simulink model "ACC_simu"  (R2023a)
settings: Solver=VariableStepAuto  StartTime=0.0  StopTime=400  RelTol=1e-3
values from neighbouring files (symbols this model uses):
  amax_ego = 1.47    [ACC_code.m]
  amin_ego = -5    [ACC_code.m]
  b = 50    [ACC_code.m]
  Brake_Pedal_Sensor = 0    [ACC_code.m]
  D_default = 10    [ACC_code.m]
  Fault_signal = 0    [ACC_code.m]
  Gas_Pedal_Sensor = 0    [ACC_code.m]
  m = 1000    [ACC_code.m]
  Time_Gap = 3    [ACC_code.m]
  Ts = 0.01    [ACC_code.m]
  v0_ego = 80    [ACC_code.m]
  v0_lead = 90    [ACC_code.m]
  x0_ego = 30    [ACC_code.m]
  x0_lead = 50    [ACC_code.m]
undefined symbols (not defined in the file or in its folder): h, km, s
libraries: aerolibconvert2 x6, simulink x2
settings Model: Creator=Leo  LastModifiedBy=Usuario
settings OptimizationCC: BlockReduction=off  DefaultParameterBehavior=Inlined  BufferReuse=off

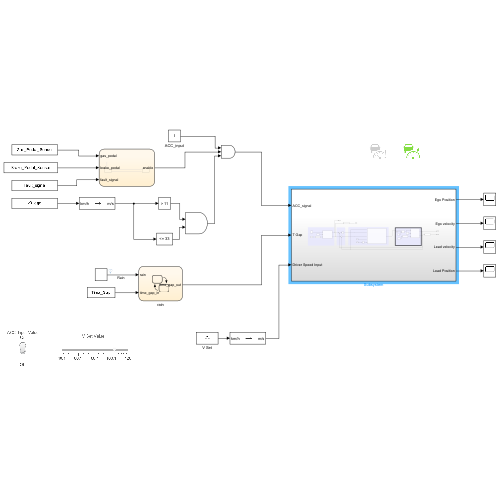
[thumbnail: Simulink's stored preview of the top-level diagram]
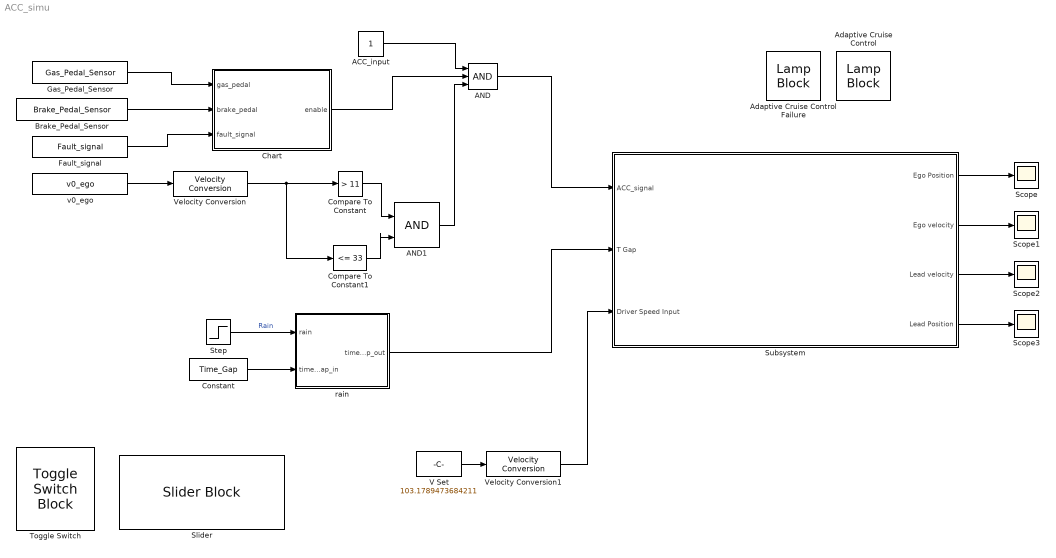
== system ACC_simu ==
  ACC_input : Constant
  AND : Logic  Inputs=3  IconShape=distinctive  AllPortsSameDT=off  OutDataTypeStr=boolean
  AND1 : Logic  IconShape=distinctive  AllPortsSameDT=off  OutDataTypeStr=boolean
  Adaptive Cruise Control : LampBlock  LabelPosition=Hide  Icon=AdaptiveCruiseControl
  Adaptive Cruise Control Failure : LampBlock  LabelPosition=Hide  Icon=AdaptiveCruiseControlFailure
  Brake_Pedal_Sensor : Constant  Value=Brake_Pedal_Sensor  SampleTime=Ts
  Chart : Stateflow chart  TreatAsAtomicUnit=on
  Compare To Constant : simulink/Logic and Bit Operations/Compare To Constant  relop=>  const=11  OutDataTypeStr=boolean
  Compare To Constant1 : simulink/Logic and Bit Operations/Compare To Constant  relop=<=  const=33  OutDataTypeStr=boolean
  Constant : Constant  Value=Time_Gap  SampleTime=Ts
  Fault_signal : Constant  Value=Fault_signal  SampleTime=Ts
  Gas_Pedal_Sensor : Constant  Value=Gas_Pedal_Sensor  SampleTime=Ts
  Scope{,1..3} (4 alike) : Scope
  Slider : SliderBlock  ScaleMin=40.1  ScaleMax=120
  Step : Step  Time=500
  Subsystem : Subsystem
  Toggle Switch : ToggleSwitchBlock
      settings: Values={{'Off', 'On'}, [0 1]}
  V Set : Constant  Value=103.1789473684211
  Velocity Conversion : aerolibconvert2/Velocity Conversion  IU=km/h  OU=m/s
  Velocity Conversion1 : aerolibconvert2/Velocity Conversion  IU=km/h  OU=m/s
  rain : Stateflow chart  TreatAsAtomicUnit=on
  v0_ego : Constant  Value=v0_ego  SampleTime=Ts
  wires:
  ACC_input/1 -> AND/1
  rain/1(time_gap_out) -> Subsystem/2(T Gap)
  Step/1 -> rain/1(rain)  "Rain"
  v0_ego/1 -> Velocity Conversion/1
  Compare To Constant/1 -> AND1/1
  Compare To Constant1/1 -> AND1/2
  AND1/1 -> AND/3
  AND/1 -> Subsystem/1(ACC_signal)
  Constant/1 -> rain/2(time_gap_in)
  Gas_Pedal_Sensor/1 -> Chart/1(gas_pedal)
  Brake_Pedal_Sensor/1 -> Chart/2(brake_pedal)
  Fault_signal/1 -> Chart/3(fault_signal)
  Chart/1(enable) -> AND/2
  Velocity Conversion/1 -> Compare To Constant1/1, Compare To Constant/1
  V Set/1 -> Velocity Conversion1/1
  Velocity Conversion1/1 -> Subsystem/3(Driver Speed Input)
  Subsystem/2(Ego velocity) -> Scope1/1
  Subsystem/1(Ego Position) -> Scope/1
  Subsystem/3(Lead velocity) -> Scope2/1
  Subsystem/4(Lead Position) -> Scope3/1

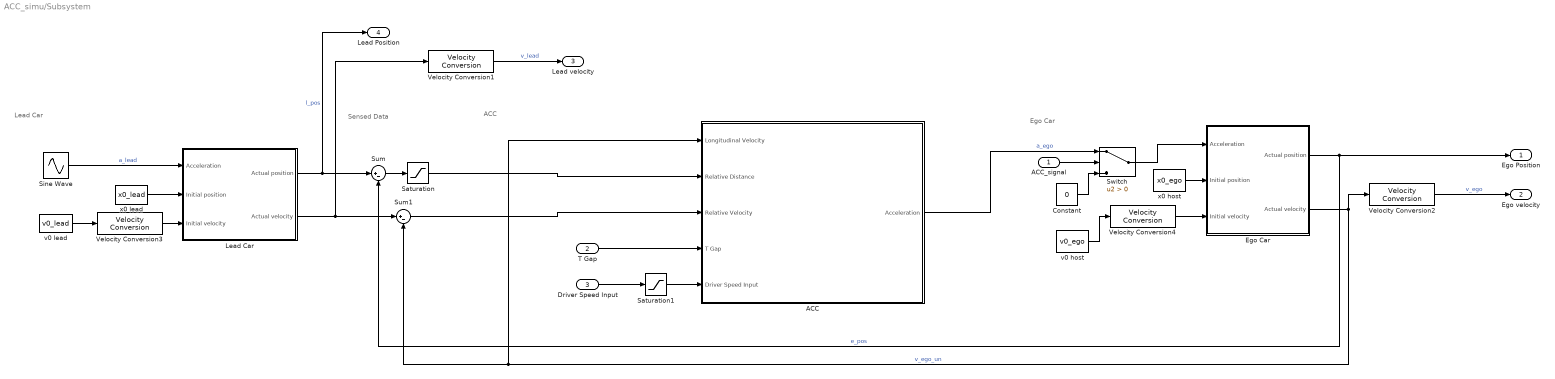
== system ACC_simu/Subsystem ==
  note: Ego Car
  note: Sensed Data
  note: Lead Car
  note: ACC
  ACC_signal : Inport
  T Gap : Inport  Port=2
  Driver Speed Input : Inport  Port=3
  ACC : Subsystem
  Constant : Constant  Value=0
  Ego Car : Subsystem
  Lead Car : Subsystem
  Saturation : Saturate  UpperLimit=200  LowerLimit=0
  Saturation1 : Saturate  UpperLimit=33  LowerLimit=11
  Sine Wave : Sin  Frequency=0.1  SampleTime=Ts
  Sum : Sum  Inputs=|+-
  Sum1 : Sum  Inputs=|+-
  Switch : Switch  Criteria=u2 > Threshold  SaturateOnIntegerOverflow=off  InputSameDT=off
  Velocity Conversion1 : aerolibconvert2/Velocity Conversion  IU=m/s  OU=km/h
  Velocity Conversion2 : aerolibconvert2/Velocity Conversion  IU=m/s  OU=km/h
  Velocity Conversion3 : aerolibconvert2/Velocity Conversion  IU=km/h  OU=m/s
  Velocity Conversion4 : aerolibconvert2/Velocity Conversion  IU=km/h  OU=m/s
  v0 host : Constant  Value=v0_ego  SampleTime=Ts
  v0 lead : Constant  Value=v0_lead  SampleTime=Ts
  x0 host : Constant  Value=x0_ego  SampleTime=Ts
  x0 lead : Constant  Value=x0_lead  SampleTime=-1
  Ego Position : Outport
  Ego velocity : Outport  Port=2
  Lead velocity : Outport  Port=3
  Lead Position : Outport  Port=4
  wires:
  v0 lead/1 -> Velocity Conversion3/1
  x0 host/1 -> Ego Car/2(Initial position)
  Ego Car/2(Actual velocity) -> Velocity Conversion2/1, ACC/1(Longitudinal Velocity), Sum1/2  "v_ego_un"
  Sum1/1 -> ACC/3(Relative Velocity)
  Ego Car/1(Actual position) -> Ego Position/1, Sum/2  "e_pos"
  Lead Car/2(Actual velocity) -> Velocity Conversion1/1, Sum1/1
  x0 lead/1 -> Lead Car/2(Initial position)
  Lead Car/1(Actual position) -> Lead Position/1, Sum/1  "l_pos"
  ACC/1(Acceleration) -> Switch/1  "a_ego"
  Sine Wave/1 -> Lead Car/1(Acceleration)  "a_lead"
  T Gap/1 -> ACC/4(T Gap)
  Sum/1 -> Saturation/1
  Saturation/1 -> ACC/2(Relative Distance)
  Switch/1 -> Ego Car/1(Acceleration)
  ACC_signal/1 -> Switch/2
  Constant/1 -> Switch/3
  Driver Speed Input/1 -> Saturation1/1
  Saturation1/1 -> ACC/5(Driver Speed Input)
  Velocity Conversion2/1 -> Ego velocity/1  "v_ego"
  Velocity Conversion1/1 -> Lead velocity/1  "v_lead"
  Velocity Conversion3/1 -> Lead Car/3(Initial velocity)
  v0 host/1 -> Velocity Conversion4/1
  Velocity Conversion4/1 -> Ego Car/3(Initial velocity)

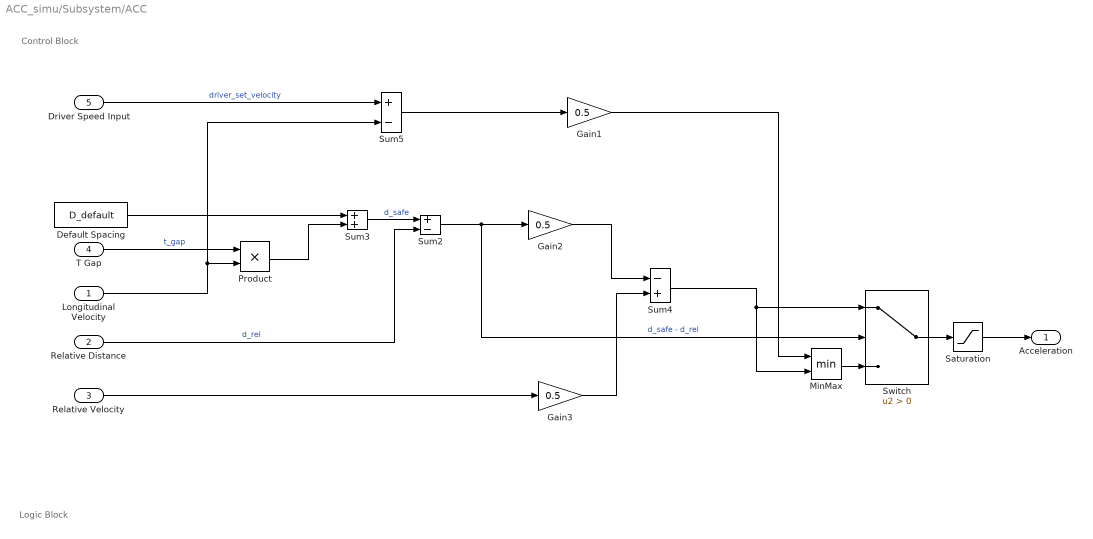
== system ACC_simu/Subsystem/ACC ==
  note: Logic Block
  note: Control Block
  Longitudinal Velocity : Inport
  Relative Distance : Inport  Port=2
  Relative Velocity : Inport  Port=3
  T Gap : Inport  Port=4
  Driver Speed Input : Inport  Port=5
  Default Spacing : Constant  Value=D_default  SampleTime=-1
  Gain1 : Gain  Gain=0.5
  Gain2 : Gain  Gain=0.5
  Gain3 : Gain  Gain=0.5
  MinMax : MinMax  Inputs=2
  Product : Product
  Saturation : Saturate  UpperLimit=amax_ego  LowerLimit=amin_ego
  Sum2 : Sum  Inputs=+-
  Sum3 : Sum
  Sum4 : Sum  Inputs=-+
  Sum5 : Sum  Inputs=+-
  Switch : Switch  Criteria=u2 > Threshold  SaturateOnIntegerOverflow=off  InputSameDT=off
  Acceleration : Outport  VectorParamsAs1DForOutWhenUnconnected=off
  wires:
  Relative Distance/1 -> Sum2/2  "d_rel"
  MinMax/1 -> Switch/3
  Switch/1 -> Saturation/1
  Driver Speed Input/1 -> Sum5/1  "driver_set_velocity"
  Gain1/1 -> MinMax/1
  Longitudinal Velocity/1 -> Product/2, Sum5/2
  Sum5/1 -> Gain1/1
  Sum2/1 -> Gain2/1, Switch/2  "d_safe - d_rel"
  Product/1 -> Sum3/2
  Gain2/1 -> Sum4/1
  Saturation/1 -> Acceleration/1
  Relative Velocity/1 -> Gain3/1
  Default Spacing/1 -> Sum3/1
  Sum3/1 -> Sum2/1  "d_safe"
  T Gap/1 -> Product/1  "t_gap"
  Sum4/1 -> MinMax/2, Switch/1
  Gain3/1 -> Sum4/2

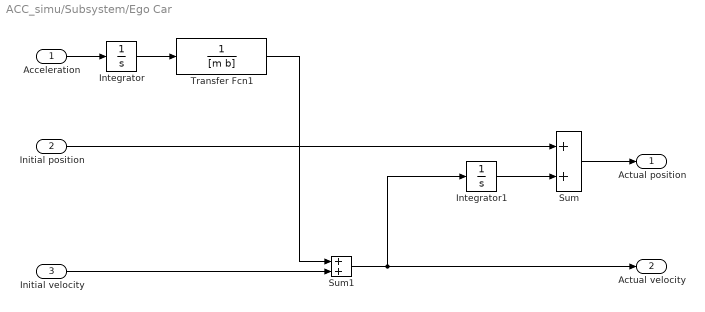
== system ACC_simu/Subsystem/Ego Car ==
  Acceleration : Inport
  Initial position : Inport  Port=2
  Initial velocity : Inport  Port=3
  Integrator : Integrator
  Integrator1 : Integrator
  Sum : Sum
  Sum1 : Sum
  Transfer Fcn1 : TransferFcn  Denominator=[m b]
  Actual position : Outport  VectorParamsAs1DForOutWhenUnconnected=off
  Actual velocity : Outport  Port=2  VectorParamsAs1DForOutWhenUnconnected=off
  wires:
  Sum1/1 -> Integrator1/1, Actual velocity/1
  Initial velocity/1 -> Sum1/2
  Sum/1 -> Actual position/1
  Transfer Fcn1/1 -> Sum1/1
  Integrator/1 -> Transfer Fcn1/1
  Acceleration/1 -> Integrator/1
  Initial position/1 -> Sum/1
  Integrator1/1 -> Sum/2

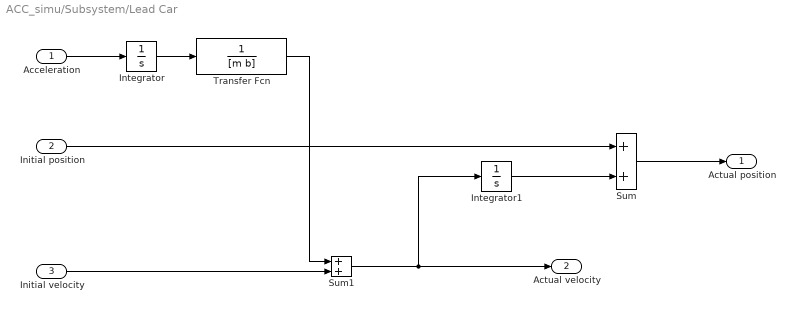
== system ACC_simu/Subsystem/Lead Car ==
  Acceleration : Inport
  Initial position : Inport  Port=2
  Initial velocity : Inport  Port=3
  Integrator : Integrator
  Integrator1 : Integrator
  Sum : Sum
  Sum1 : Sum
  Transfer Fcn : TransferFcn  Denominator=[m b]
  Actual position : Outport  VectorParamsAs1DForOutWhenUnconnected=off
  Actual velocity : Outport  Port=2  VectorParamsAs1DForOutWhenUnconnected=off
  wires:
  Transfer Fcn/1 -> Sum1/1
  Initial velocity/1 -> Sum1/2
  Sum/1 -> Actual position/1
  Integrator/1 -> Transfer Fcn/1
  Sum1/1 -> Integrator1/1, Actual velocity/1
  Initial position/1 -> Sum/1
  Integrator1/1 -> Sum/2
  Acceleration/1 -> Integrator/1

== stateflow chart ACC_simu/rain ==
  state no_rain
    entry:
    time_gap_out = time_gap_in
  state rain
    entry:
    time_gap_out = 2*time_gap_in
  (default) -> no_rain
  no_rain -> rain : [rain == 1]
  rain -> no_rain : [rain == 0]
  data: rain input; time_gap_out output; time_gap_in input

== stateflow chart ACC_simu/Chart ==
  state Operational
    entry:
    enable = 1;
  state Disable
    entry:
    enable = 0;
  (default) -> Operational
  Disable -> Operational : [gas_pedal == 0 && brake_pedal == 0 && fault_signal == 0]
  Operational -> Disable : [gas_pedal == 1 || brake_pedal == 1 || fault_signal == 1]
  data: gas_pedal input; brake_pedal input; enable output; fault_signal input
